simulink model "Fahrwiderstandsgleichung_2016a"  (R2016a)
settings: Solver=ode4  SolverMode=SingleTasking  StartTime=0.0  StopTime=100  RelTol=1e-3
values from neighbouring files (symbols this model uses):
  A = 2.51    [Uebung_Jingsheng.m]
  c_w = 0.33    [Uebung_Jingsheng.m]
  dkv_lookup = [0 0.2 0.3 0.4 0.5 0.6 0.7 0.8 0.9 1]    [Motorkennfeld.mat]
  g = 9.81    [Uebung_Jingsheng.m]
  i_D = 3.684    [Uebung_Jingsheng.m]
  i_G = 2.22    [Uebung_Jingsheng.m]
  k_r = 0.015    [Uebung_Jingsheng.m]
  m = 1770    [Uebung_Jingsheng.m]
  M_mot_m_lookup = [0 35.055422338 52.583133507 70.110844676 87.638555845 105.166267014 122.693978183 140.221689352 157.749400521 175.27711169 0 57.1760081386 ... (60 elements, 10x6)]    [Motorkennfeld.mat]
  m_rot = 48.3    [Uebung_Jingsheng.m]
  q = 0.3    [Uebung_Jingsheng.m]
  r = 0.33    [Uebung_Jingsheng.m]
  roh = 1.22    [Uebung_Jingsheng.m]
  w_all_m_lookup = [105.883191599 151.789190651 209.70026243 316.859987844 422.642648478 473.041125024]    [Motorkennfeld.mat]
settings Model: Creator=Jason  LastModifiedBy=Jason
settings DebuggingCC: SFUnexpectedBacktrackingDiag=error  SFNoUnconditionalDefaultTransitionDiag=error
settings GRTTargetCC: TargetLangStandard=C99 (ISO)  GeneratePreprocessorConditionals=Use local settings
settings ConfigComp: CovMetricSettings=dwe  CovHtmlReporting=off  CovSaveCumulativeToWorkspaceVar=off  CovSaveSingleToWorkspaceVar=off  CovExternalEMLEnable=on

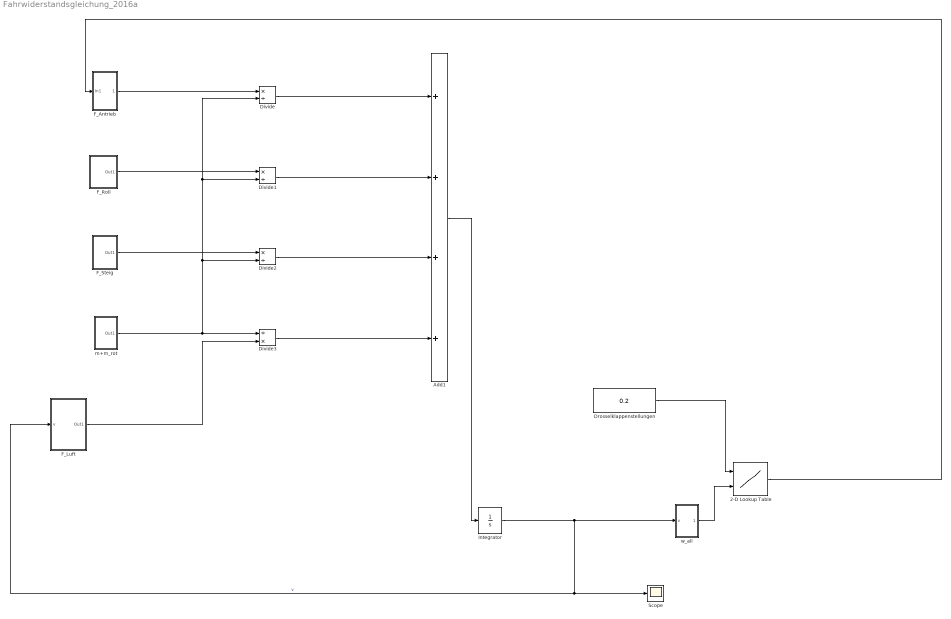
== system Fahrwiderstandsgleichung_2016a ==
  " Drosselklappenstellungen " : Constant  Value=0.2
  2-D Lookup Table : Lookup_n-D  BreakpointsForDimension1=dkv_lookup  BreakpointsForDimension2=w_all_m_lookup  Table=M_mot_m_lookup  InternalRulePriority=Speed  RndMeth=Simplest  InputSameDT=on
  Add1 : Sum  Inputs=++++
  Divide : Product  Inputs=*/
  Divide1 : Product  Inputs=*/
  Divide2 : Product  Inputs=*/
  Divide3 : Product  Inputs=/*
  F_Antrieb : Subsystem
  F_Luft : Subsystem
  F_Roll : Subsystem
  F_Steig : Subsystem
  Integrator : Integrator  InitialCondition=10
  Scope : Scope
  m+m_rot : Subsystem
  w_all : Subsystem
  wires:
  Integrator/1 -> F_Luft/1(v), Scope/1, w_all/1(v)  "v"
  " Drosselklappenstellungen "/1 -> 2-D Lookup Table/1
  Divide/1 -> Add1/1
  Divide1/1 -> Add1/2
  Divide2/1 -> Add1/3
  Add1/1 -> Integrator/1
  Divide3/1 -> Add1/4
  F_Steig/1(Out1) -> Divide2/1
  F_Roll/1(Out1) -> Divide1/1
  m+m_rot/1(Out1) -> Divide/2, Divide1/2, Divide2/2, Divide3/1
  w_all/1(Out1) -> 2-D Lookup Table/2
  F_Luft/1(Out1) -> Divide3/2
  2-D Lookup Table/1 -> F_Antrieb/1(In1)
  F_Antrieb/1(Out1) -> Divide/1

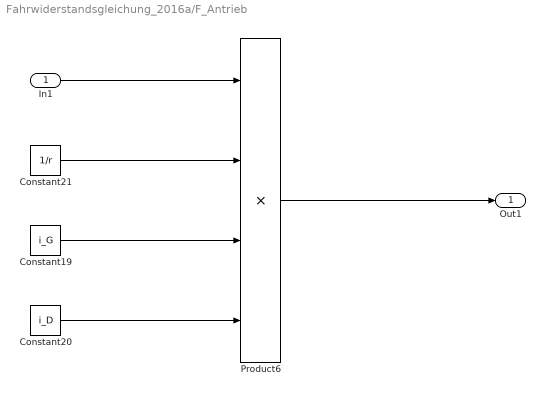
== system Fahrwiderstandsgleichung_2016a/F_Antrieb ==
  In1 : Inport
  Constant19 : Constant  Value=i_G
  Constant20 : Constant  Value=i_D
  Constant21 : Constant  Value=1/r
  Product6 : Product  Inputs=4
  Out1 : Outport
  wires:
  Constant20/1 -> Product6/4
  In1/1 -> Product6/1
  Constant19/1 -> Product6/3
  Product6/1 -> Out1/1
  Constant21/1 -> Product6/2

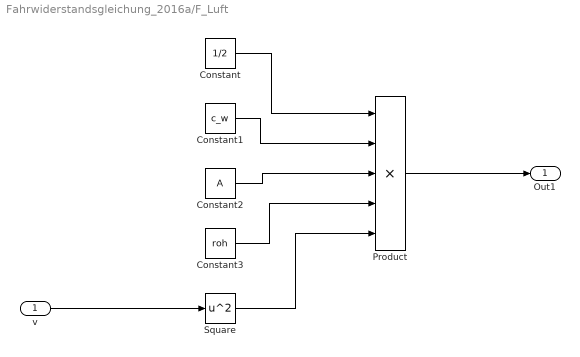
== system Fahrwiderstandsgleichung_2016a/F_Luft ==
  v : Inport
  Constant : Constant  Value=1/2
  Constant1 : Constant  Value=c_w
  Constant2 : Constant  Value=A
  Constant3 : Constant  Value=roh
  Product : Product  Inputs=5
  Square : Math  Operator=square  SaturateOnIntegerOverflow=on
  Out1 : Outport
  wires:
  Constant/1 -> Product/1
  Constant3/1 -> Product/4
  Constant2/1 -> Product/3
  v/1 -> Square/1
  Constant1/1 -> Product/2
  Product/1 -> Out1/1
  Square/1 -> Product/5

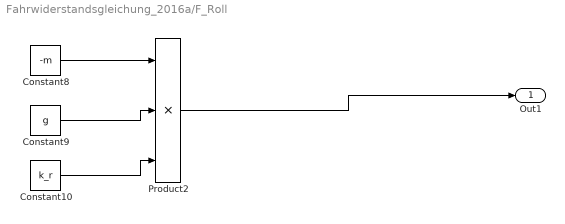
== system Fahrwiderstandsgleichung_2016a/F_Roll ==
  Constant10 : Constant  Value=k_r
  Constant8 : Constant  Value=-m
  Constant9 : Constant  Value=g
  Product2 : Product  Inputs=3
  Out1 : Outport
  wires:
  Constant9/1 -> Product2/2
  Product2/1 -> Out1/1
  Constant8/1 -> Product2/1
  Constant10/1 -> Product2/3

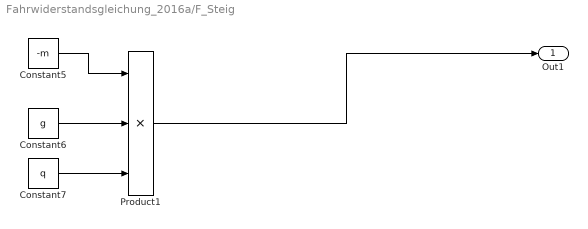
== system Fahrwiderstandsgleichung_2016a/F_Steig ==
  Constant5 : Constant  Value=-m
  Constant6 : Constant  Value=g
  Constant7 : Constant  Value=q
  Product1 : Product  Inputs=3
  Out1 : Outport
  wires:
  Product1/1 -> Out1/1
  Constant6/1 -> Product1/2
  Constant5/1 -> Product1/1
  Constant7/1 -> Product1/3

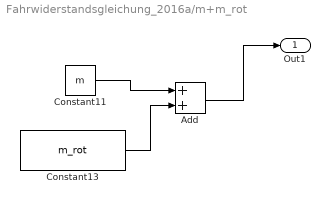
== system Fahrwiderstandsgleichung_2016a/m+m_rot ==
  Add : Sum
  Constant11 : Constant  Value=m
  Constant13 : Constant  Value=m_rot
  Out1 : Outport
  wires:
  Constant13/1 -> Add/2
  Constant11/1 -> Add/1
  Add/1 -> Out1/1

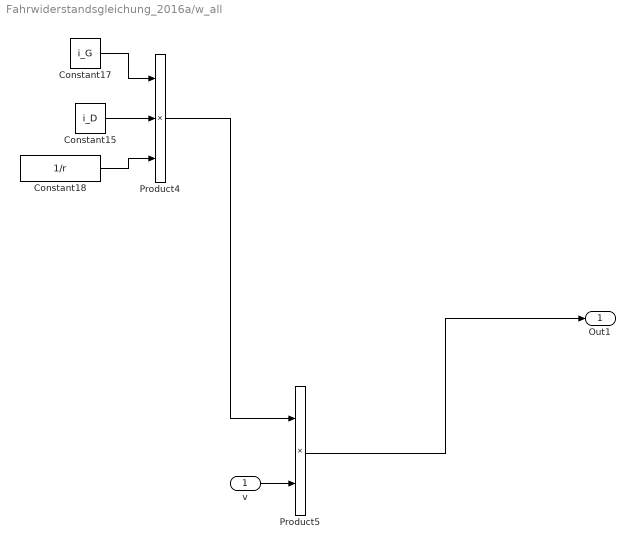
== system Fahrwiderstandsgleichung_2016a/w_all ==
  v : Inport
  Constant15 : Constant  Value=i_D
  Constant17 : Constant  Value=i_G
  Constant18 : Constant  Value=1/r
  Product4 : Product  Inputs=3
  Product5 : Product
  Out1 : Outport
  wires:
  Product4/1 -> Product5/1
  Constant17/1 -> Product4/1
  Constant18/1 -> Product4/3
  Product5/1 -> Out1/1
  Constant15/1 -> Product4/2
  v/1 -> Product5/2
